simulink model "qless_forgetting_factor_16x16_nofifo"  (R2021a)
settings: Solver=FixedStepDiscrete  StartTime=0.0  StopTime=stoptime*inf  RelTol=1e-3
InitFcn:
  | qless_init_16chan_fi
undefined symbols (not defined in the file): fc, numArrayElements, physconst, srcAngles, Ts
libraries: hdlsllib x137, commfilt2 x4, commrfcorlib x3, commsync2 x3, commrflib2 x2, commrandsrc3 x2, simulink x2, phasedtxrxlib x2, commdigbbndcpm2 x1, embreciprocals x1, commdigbbndpm3 x1
(part 9 of 22)

== system qless_forgetting_factor_16x16_nofifo/MVDR_QLess_HDL/Complex Partial-Systolic Matrix Solve Using Q-less QR Decomposition with Forgetting Factor Manually Tiled n=16/Complex Partial-Systolic Q-less QR with Forgetting Factor/Complex Partial-Systolic Q-less QR with Forgetting Factor Manually tiled/Complex Partial-Systolic Q-less QR Decomposition with Forgetting Factor Section Constant pivot3/Complex Partial-Systolic Q-less QR Row Rotations/ValidIn to Ready Logic1 ==
  readyIn : Inport
  validIn : Inport  Port=2
  AND : Logic  IconShape=distinctive  AllPortsSameDT=off  OutDataTypeStr=boolean
  NOT : Logic  Operator=NOT  IconShape=distinctive  AllPortsSameDT=off  OutDataTypeStr=boolean
  readyOut : Outport  VectorParamsAs1DForOutWhenUnconnected=off
  wires:
  validIn/1 -> NOT/1
  readyIn/1 -> AND/1
  AND/1 -> readyOut/1
  NOT/1 -> AND/2

== system qless_forgetting_factor_16x16_nofifo/MVDR_QLess_HDL/Complex Partial-Systolic Matrix Solve Using Q-less QR Decomposition with Forgetting Factor Manually Tiled n=16/Complex Partial-Systolic Q-less QR with Forgetting Factor/Complex Partial-Systolic Q-less QR with Forgetting Factor Manually tiled/Complex Partial-Systolic Q-less QR Decomposition with Forgetting Factor Section Constant pivot4/Complex Partial-Systolic Q-less QR Row Rotations/Complex Partial-Systolic Q-less QR CORDIC Row Rotation ==
  x : Inport
  y : Inport  Port=2
  validIn : Inport  Port=3
  restart : Inport  Port=4
  CORDIC QR Kernel : MATLAB Function  TreatAsAtomicUnit=on
  Delay{1..3,6} (4 alike) : Delay  DelayLength=1
  State Control : StateControl  StateControl=Synchronous
  Unit Delay Enabled Synchronous1 : hdlsllib/Discrete/Unit Delay Enabled Synchronous  InitialCondition=0.0  SampleTime=-1
      settings: SourceProductBaseCode=SL
  Unit Delay Enabled Synchronous4 : hdlsllib/Discrete/Unit Delay Enabled Synchronous  InitialCondition=0.0  SampleTime=-1
      settings: SourceProductBaseCode=SL
  xOut : Outport  VectorParamsAs1DForOutWhenUnconnected=off
  yOut : Outport  Port=2  VectorParamsAs1DForOutWhenUnconnected=off
  validOut : Outport  Port=3  VectorParamsAs1DForOutWhenUnconnected=off
  ready : Outport  Port=4  VectorParamsAs1DForOutWhenUnconnected=off
  wires:
  Delay3/1 -> validOut/1
  Unit Delay Enabled Synchronous1/1 -> yOut/1
  CORDIC QR Kernel/1(xOut) -> Unit Delay Enabled Synchronous4/1
  y/1 -> Delay2/1
  x/1 -> Delay1/1
  CORDIC QR Kernel/2(yOut) -> Unit Delay Enabled Synchronous1/1
  validIn/1 -> Delay6/1
  Unit Delay Enabled Synchronous4/1 -> xOut/1
  restart/1 -> CORDIC QR Kernel/4(restart)
  CORDIC QR Kernel/3(validOut) -> Delay3/1, Unit Delay Enabled Synchronous4/2, Unit Delay Enabled Synchronous1/2
  CORDIC QR Kernel/4(ready) -> ready/1
  Delay1/1 -> CORDIC QR Kernel/1(xIn)
  Delay2/1 -> CORDIC QR Kernel/2(yIn)
  Delay6/1 -> CORDIC QR Kernel/3(validIn)

== system qless_forgetting_factor_16x16_nofifo/MVDR_QLess_HDL/Complex Partial-Systolic Matrix Solve Using Q-less QR Decomposition with Forgetting Factor Manually Tiled n=16/Complex Partial-Systolic Q-less QR with Forgetting Factor/Complex Partial-Systolic Q-less QR with Forgetting Factor Manually tiled/Complex Partial-Systolic Q-less QR Decomposition with Forgetting Factor Section Constant pivot4/Complex Partial-Systolic Q-less QR Row Rotations/Inverse CORDIC Gain1 ==
  u : Inport
  MATLAB Function : MATLAB Function  TreatAsAtomicUnit=on
  y : Outport  VectorParamsAs1DForOutWhenUnconnected=off
  wires:
  MATLAB Function/1(y) -> y/1
  u/1 -> MATLAB Function/1(u)

== system qless_forgetting_factor_16x16_nofifo/MVDR_QLess_HDL/Complex Partial-Systolic Matrix Solve Using Q-less QR Decomposition with Forgetting Factor Manually Tiled n=16/Complex Partial-Systolic Q-less QR with Forgetting Factor/Complex Partial-Systolic Q-less QR with Forgetting Factor Manually tiled/Complex Partial-Systolic Q-less QR Decomposition with Forgetting Factor Section Constant pivot4/Complex Partial-Systolic Q-less QR Row Rotations/Inverse CORDIC Gain4 ==
  u : Inport
  MATLAB Function : MATLAB Function  TreatAsAtomicUnit=on
  y : Outport  VectorParamsAs1DForOutWhenUnconnected=off
  wires:
  MATLAB Function/1(y) -> y/1
  u/1 -> MATLAB Function/1(u)

== system qless_forgetting_factor_16x16_nofifo/MVDR_QLess_HDL/Complex Partial-Systolic Matrix Solve Using Q-less QR Decomposition with Forgetting Factor Manually Tiled n=16/Complex Partial-Systolic Q-less QR with Forgetting Factor/Complex Partial-Systolic Q-less QR with Forgetting Factor Manually tiled/Complex Partial-Systolic Q-less QR Decomposition with Forgetting Factor Section Constant pivot4/Complex Partial-Systolic Q-less QR Row Rotations/Q-less QR Rotate First Element To Real1 ==
  x : Inport
  validIn : Inport  Port=2
  restart : Inport  Port=3
  Complex to Real-Imag : ComplexToRealImag
  Delay15 : Delay  DelayLength=1
  Delay9 : Delay  DelayLength=1
  Q-less QR Real Row Rotations : Subsystem  mask(QR Real Row Rotations){n=n, pivot=pivot}
      mask prompts: n "fixed:emblib:ColumnsInA"
      mask help: fixed:emblib:RowRotationsFullDescription
      mask DialogControl n Prompt: Number of columns in matrix A
  Real-Imag to Complex : RealImagToComplex
  State Control : StateControl  StateControl=Synchronous
  Unit Delay Enabled Synchronous1 : hdlsllib/Discrete/Unit Delay Enabled Synchronous  InitialCondition=0.0  SampleTime=-1
      settings: SourceProductBaseCode=SL
  Unit Delay Enabled Synchronous3 : hdlsllib/Discrete/Unit Delay Enabled Synchronous  InitialCondition=0.0  SampleTime=-1
      settings: SourceProductBaseCode=SL
  ValidIn to Ready Logic : Subsystem
  ValidIn to Ready Logic1 : Subsystem
  xOut : Outport  VectorParamsAs1DForOutWhenUnconnected=off
  validOut : Outport  Port=2  VectorParamsAs1DForOutWhenUnconnected=off
  ready : Outport  Port=3  VectorParamsAs1DForOutWhenUnconnected=off
  wires:
  Q-less QR Real Row Rotations/2(yOut) -> Real-Imag to Complex/2
  Q-less QR Real Row Rotations/1(xOut) -> Real-Imag to Complex/1
  Complex to Real-Imag/2 -> Q-less QR Real Row Rotations/2(y)
  Complex to Real-Imag/1 -> Q-less QR Real Row Rotations/1(x)
  restart/1 -> Q-less QR Real Row Rotations/4(restart)
  ValidIn to Ready Logic1/1(readyOut) -> ready/1
  ValidIn to Ready Logic/1(readyOut) -> ValidIn to Ready Logic1/1(readyIn)
  Q-less QR Real Row Rotations/4(ready) -> ValidIn to Ready Logic/1(readyIn)
  Q-less QR Real Row Rotations/3(validOut) -> Delay15/1, Unit Delay Enabled Synchronous3/2
  Delay9/1 -> ValidIn to Ready Logic/2(validIn), Q-less QR Real Row Rotations/3(validIn)
  x/1 -> Unit Delay Enabled Synchronous1/1
  validIn/1 -> ValidIn to Ready Logic1/2(validIn), Delay9/1, Unit Delay Enabled Synchronous1/2
  Delay15/1 -> validOut/1
  Unit Delay Enabled Synchronous1/1 -> Complex to Real-Imag/1
  Real-Imag to Complex/1 -> Unit Delay Enabled Synchronous3/1
  Unit Delay Enabled Synchronous3/1 -> xOut/1

== system qless_forgetting_factor_16x16_nofifo/MVDR_QLess_HDL/Complex Partial-Systolic Matrix Solve Using Q-less QR Decomposition with Forgetting Factor Manually Tiled n=16/Complex Partial-Systolic Q-less QR with Forgetting Factor/Complex Partial-Systolic Q-less QR with Forgetting Factor Manually tiled/Complex Partial-Systolic Q-less QR Decomposition with Forgetting Factor Section Constant pivot4/Complex Partial-Systolic Q-less QR Row Rotations/Set Element To Zero1 ==
  u : Inport
  Set Element To Zero : MATLAB Function  TreatAsAtomicUnit=on
  y : Outport  VectorParamsAs1DForOutWhenUnconnected=off
  wires:
  Set Element To Zero/1(y) -> y/1
  u/1 -> Set Element To Zero/1(u)

== system qless_forgetting_factor_16x16_nofifo/MVDR_QLess_HDL/Complex Partial-Systolic Matrix Solve Using Q-less QR Decomposition with Forgetting Factor Manually Tiled n=16/Complex Partial-Systolic Q-less QR with Forgetting Factor/Complex Partial-Systolic Q-less QR with Forgetting Factor Manually tiled/Complex Partial-Systolic Q-less QR Decomposition with Forgetting Factor Section Constant pivot4/Complex Partial-Systolic Q-less QR Row Rotations/ValidIn to Ready Logic ==
  readyIn : Inport
  validIn : Inport  Port=2
  AND : Logic  IconShape=distinctive  AllPortsSameDT=off  OutDataTypeStr=boolean
  NOT : Logic  Operator=NOT  IconShape=distinctive  AllPortsSameDT=off  OutDataTypeStr=boolean
  readyOut : Outport  VectorParamsAs1DForOutWhenUnconnected=off
  wires:
  validIn/1 -> NOT/1
  readyIn/1 -> AND/1
  AND/1 -> readyOut/1
  NOT/1 -> AND/2

== system qless_forgetting_factor_16x16_nofifo/MVDR_QLess_HDL/Complex Partial-Systolic Matrix Solve Using Q-less QR Decomposition with Forgetting Factor Manually Tiled n=16/Complex Partial-Systolic Q-less QR with Forgetting Factor/Complex Partial-Systolic Q-less QR with Forgetting Factor Manually tiled/Complex Partial-Systolic Q-less QR Decomposition with Forgetting Factor Section Constant pivot4/Complex Partial-Systolic Q-less QR Row Rotations/ValidIn to Ready Logic1 ==
  readyIn : Inport
  validIn : Inport  Port=2
  AND : Logic  IconShape=distinctive  AllPortsSameDT=off  OutDataTypeStr=boolean
  NOT : Logic  Operator=NOT  IconShape=distinctive  AllPortsSameDT=off  OutDataTypeStr=boolean
  readyOut : Outport  VectorParamsAs1DForOutWhenUnconnected=off
  wires:
  validIn/1 -> NOT/1
  readyIn/1 -> AND/1
  AND/1 -> readyOut/1
  NOT/1 -> AND/2

== system qless_forgetting_factor_16x16_nofifo/MVDR_QLess_HDL/Complex Partial-Systolic Matrix Solve Using Q-less QR Decomposition with Forgetting Factor Manually Tiled n=16/Complex Partial-Systolic Q-less QR with Forgetting Factor/Complex Partial-Systolic Q-less QR with Forgetting Factor Manually tiled/Complex Partial-Systolic Q-less QR Decomposition with Forgetting Factor Section Constant pivot5/Complex Partial-Systolic Q-less QR Row Rotations/Complex Partial-Systolic Q-less QR CORDIC Row Rotation ==
  x : Inport
  y : Inport  Port=2
  validIn : Inport  Port=3
  restart : Inport  Port=4
  CORDIC QR Kernel : MATLAB Function  TreatAsAtomicUnit=on
  Delay{1..3,6} (4 alike) : Delay  DelayLength=1
  State Control : StateControl  StateControl=Synchronous
  Unit Delay Enabled Synchronous1 : hdlsllib/Discrete/Unit Delay Enabled Synchronous  InitialCondition=0.0  SampleTime=-1
      settings: SourceProductBaseCode=SL
  Unit Delay Enabled Synchronous4 : hdlsllib/Discrete/Unit Delay Enabled Synchronous  InitialCondition=0.0  SampleTime=-1
      settings: SourceProductBaseCode=SL
  xOut : Outport  VectorParamsAs1DForOutWhenUnconnected=off
  yOut : Outport  Port=2  VectorParamsAs1DForOutWhenUnconnected=off
  validOut : Outport  Port=3  VectorParamsAs1DForOutWhenUnconnected=off
  ready : Outport  Port=4  VectorParamsAs1DForOutWhenUnconnected=off
  wires:
  Delay3/1 -> validOut/1
  Unit Delay Enabled Synchronous1/1 -> yOut/1
  CORDIC QR Kernel/1(xOut) -> Unit Delay Enabled Synchronous4/1
  y/1 -> Delay2/1
  x/1 -> Delay1/1
  CORDIC QR Kernel/2(yOut) -> Unit Delay Enabled Synchronous1/1
  validIn/1 -> Delay6/1
  Unit Delay Enabled Synchronous4/1 -> xOut/1
  restart/1 -> CORDIC QR Kernel/4(restart)
  CORDIC QR Kernel/3(validOut) -> Delay3/1, Unit Delay Enabled Synchronous4/2, Unit Delay Enabled Synchronous1/2
  CORDIC QR Kernel/4(ready) -> ready/1
  Delay1/1 -> CORDIC QR Kernel/1(xIn)
  Delay2/1 -> CORDIC QR Kernel/2(yIn)
  Delay6/1 -> CORDIC QR Kernel/3(validIn)

== system qless_forgetting_factor_16x16_nofifo/MVDR_QLess_HDL/Complex Partial-Systolic Matrix Solve Using Q-less QR Decomposition with Forgetting Factor Manually Tiled n=16/Complex Partial-Systolic Q-less QR with Forgetting Factor/Complex Partial-Systolic Q-less QR with Forgetting Factor Manually tiled/Complex Partial-Systolic Q-less QR Decomposition with Forgetting Factor Section Constant pivot5/Complex Partial-Systolic Q-less QR Row Rotations/Inverse CORDIC Gain1 ==
  u : Inport
  MATLAB Function : MATLAB Function  TreatAsAtomicUnit=on
  y : Outport  VectorParamsAs1DForOutWhenUnconnected=off
  wires:
  MATLAB Function/1(y) -> y/1
  u/1 -> MATLAB Function/1(u)

== system qless_forgetting_factor_16x16_nofifo/MVDR_QLess_HDL/Complex Partial-Systolic Matrix Solve Using Q-less QR Decomposition with Forgetting Factor Manually Tiled n=16/Complex Partial-Systolic Q-less QR with Forgetting Factor/Complex Partial-Systolic Q-less QR with Forgetting Factor Manually tiled/Complex Partial-Systolic Q-less QR Decomposition with Forgetting Factor Section Constant pivot5/Complex Partial-Systolic Q-less QR Row Rotations/Inverse CORDIC Gain4 ==
  u : Inport
  MATLAB Function : MATLAB Function  TreatAsAtomicUnit=on
  y : Outport  VectorParamsAs1DForOutWhenUnconnected=off
  wires:
  MATLAB Function/1(y) -> y/1
  u/1 -> MATLAB Function/1(u)

== system qless_forgetting_factor_16x16_nofifo/MVDR_QLess_HDL/Complex Partial-Systolic Matrix Solve Using Q-less QR Decomposition with Forgetting Factor Manually Tiled n=16/Complex Partial-Systolic Q-less QR with Forgetting Factor/Complex Partial-Systolic Q-less QR with Forgetting Factor Manually tiled/Complex Partial-Systolic Q-less QR Decomposition with Forgetting Factor Section Constant pivot5/Complex Partial-Systolic Q-less QR Row Rotations/Q-less QR Rotate First Element To Real1 ==
  x : Inport
  validIn : Inport  Port=2
  restart : Inport  Port=3
  Complex to Real-Imag : ComplexToRealImag
  Delay15 : Delay  DelayLength=1
  Delay9 : Delay  DelayLength=1
  Q-less QR Real Row Rotations : Subsystem  mask(QR Real Row Rotations){n=n, pivot=pivot}
      mask prompts: n "fixed:emblib:ColumnsInA"
      mask help: fixed:emblib:RowRotationsFullDescription
      mask DialogControl n Prompt: Number of columns in matrix A
  Real-Imag to Complex : RealImagToComplex
  State Control : StateControl  StateControl=Synchronous
  Unit Delay Enabled Synchronous1 : hdlsllib/Discrete/Unit Delay Enabled Synchronous  InitialCondition=0.0  SampleTime=-1
      settings: SourceProductBaseCode=SL
  Unit Delay Enabled Synchronous3 : hdlsllib/Discrete/Unit Delay Enabled Synchronous  InitialCondition=0.0  SampleTime=-1
      settings: SourceProductBaseCode=SL
  ValidIn to Ready Logic : Subsystem
  ValidIn to Ready Logic1 : Subsystem
  xOut : Outport  VectorParamsAs1DForOutWhenUnconnected=off
  validOut : Outport  Port=2  VectorParamsAs1DForOutWhenUnconnected=off
  ready : Outport  Port=3  VectorParamsAs1DForOutWhenUnconnected=off
  wires:
  Q-less QR Real Row Rotations/2(yOut) -> Real-Imag to Complex/2
  Q-less QR Real Row Rotations/1(xOut) -> Real-Imag to Complex/1
  Complex to Real-Imag/2 -> Q-less QR Real Row Rotations/2(y)
  Complex to Real-Imag/1 -> Q-less QR Real Row Rotations/1(x)
  restart/1 -> Q-less QR Real Row Rotations/4(restart)
  ValidIn to Ready Logic1/1(readyOut) -> ready/1
  ValidIn to Ready Logic/1(readyOut) -> ValidIn to Ready Logic1/1(readyIn)
  Q-less QR Real Row Rotations/4(ready) -> ValidIn to Ready Logic/1(readyIn)
  Q-less QR Real Row Rotations/3(validOut) -> Delay15/1, Unit Delay Enabled Synchronous3/2
  Delay9/1 -> ValidIn to Ready Logic/2(validIn), Q-less QR Real Row Rotations/3(validIn)
  x/1 -> Unit Delay Enabled Synchronous1/1
  validIn/1 -> ValidIn to Ready Logic1/2(validIn), Delay9/1, Unit Delay Enabled Synchronous1/2
  Delay15/1 -> validOut/1
  Unit Delay Enabled Synchronous1/1 -> Complex to Real-Imag/1
  Real-Imag to Complex/1 -> Unit Delay Enabled Synchronous3/1
  Unit Delay Enabled Synchronous3/1 -> xOut/1

== system qless_forgetting_factor_16x16_nofifo/MVDR_QLess_HDL/Complex Partial-Systolic Matrix Solve Using Q-less QR Decomposition with Forgetting Factor Manually Tiled n=16/Complex Partial-Systolic Q-less QR with Forgetting Factor/Complex Partial-Systolic Q-less QR with Forgetting Factor Manually tiled/Complex Partial-Systolic Q-less QR Decomposition with Forgetting Factor Section Constant pivot5/Complex Partial-Systolic Q-less QR Row Rotations/Set Element To Zero1 ==
  u : Inport
  Set Element To Zero : MATLAB Function  TreatAsAtomicUnit=on
  y : Outport  VectorParamsAs1DForOutWhenUnconnected=off
  wires:
  Set Element To Zero/1(y) -> y/1
  u/1 -> Set Element To Zero/1(u)

== system qless_forgetting_factor_16x16_nofifo/MVDR_QLess_HDL/Complex Partial-Systolic Matrix Solve Using Q-less QR Decomposition with Forgetting Factor Manually Tiled n=16/Complex Partial-Systolic Q-less QR with Forgetting Factor/Complex Partial-Systolic Q-less QR with Forgetting Factor Manually tiled/Complex Partial-Systolic Q-less QR Decomposition with Forgetting Factor Section Constant pivot5/Complex Partial-Systolic Q-less QR Row Rotations/ValidIn to Ready Logic ==
  readyIn : Inport
  validIn : Inport  Port=2
  AND : Logic  IconShape=distinctive  AllPortsSameDT=off  OutDataTypeStr=boolean
  NOT : Logic  Operator=NOT  IconShape=distinctive  AllPortsSameDT=off  OutDataTypeStr=boolean
  readyOut : Outport  VectorParamsAs1DForOutWhenUnconnected=off
  wires:
  validIn/1 -> NOT/1
  readyIn/1 -> AND/1
  AND/1 -> readyOut/1
  NOT/1 -> AND/2

== system qless_forgetting_factor_16x16_nofifo/MVDR_QLess_HDL/Complex Partial-Systolic Matrix Solve Using Q-less QR Decomposition with Forgetting Factor Manually Tiled n=16/Complex Partial-Systolic Q-less QR with Forgetting Factor/Complex Partial-Systolic Q-less QR with Forgetting Factor Manually tiled/Complex Partial-Systolic Q-less QR Decomposition with Forgetting Factor Section Constant pivot5/Complex Partial-Systolic Q-less QR Row Rotations/ValidIn to Ready Logic1 ==
  readyIn : Inport
  validIn : Inport  Port=2
  AND : Logic  IconShape=distinctive  AllPortsSameDT=off  OutDataTypeStr=boolean
  NOT : Logic  Operator=NOT  IconShape=distinctive  AllPortsSameDT=off  OutDataTypeStr=boolean
  readyOut : Outport  VectorParamsAs1DForOutWhenUnconnected=off
  wires:
  validIn/1 -> NOT/1
  readyIn/1 -> AND/1
  AND/1 -> readyOut/1
  NOT/1 -> AND/2

== system qless_forgetting_factor_16x16_nofifo/MVDR_QLess_HDL/Complex Partial-Systolic Matrix Solve Using Q-less QR Decomposition with Forgetting Factor Manually Tiled n=16/Complex Partial-Systolic Q-less QR with Forgetting Factor/Complex Partial-Systolic Q-less QR with Forgetting Factor Manually tiled/Complex Partial-Systolic Q-less QR Decomposition with Forgetting Factor Section Constant pivot6/Complex Partial-Systolic Q-less QR Row Rotations/Complex Partial-Systolic Q-less QR CORDIC Row Rotation ==
  x : Inport
  y : Inport  Port=2
  validIn : Inport  Port=3
  restart : Inport  Port=4
  CORDIC QR Kernel : MATLAB Function  TreatAsAtomicUnit=on
  Delay{1..3,6} (4 alike) : Delay  DelayLength=1
  State Control : StateControl  StateControl=Synchronous
  Unit Delay Enabled Synchronous1 : hdlsllib/Discrete/Unit Delay Enabled Synchronous  InitialCondition=0.0  SampleTime=-1
      settings: SourceProductBaseCode=SL
  Unit Delay Enabled Synchronous4 : hdlsllib/Discrete/Unit Delay Enabled Synchronous  InitialCondition=0.0  SampleTime=-1
      settings: SourceProductBaseCode=SL
  xOut : Outport  VectorParamsAs1DForOutWhenUnconnected=off
  yOut : Outport  Port=2  VectorParamsAs1DForOutWhenUnconnected=off
  validOut : Outport  Port=3  VectorParamsAs1DForOutWhenUnconnected=off
  ready : Outport  Port=4  VectorParamsAs1DForOutWhenUnconnected=off
  wires:
  Delay3/1 -> validOut/1
  Unit Delay Enabled Synchronous1/1 -> yOut/1
  CORDIC QR Kernel/1(xOut) -> Unit Delay Enabled Synchronous4/1
  y/1 -> Delay2/1
  x/1 -> Delay1/1
  CORDIC QR Kernel/2(yOut) -> Unit Delay Enabled Synchronous1/1
  validIn/1 -> Delay6/1
  Unit Delay Enabled Synchronous4/1 -> xOut/1
  restart/1 -> CORDIC QR Kernel/4(restart)
  CORDIC QR Kernel/3(validOut) -> Delay3/1, Unit Delay Enabled Synchronous4/2, Unit Delay Enabled Synchronous1/2
  CORDIC QR Kernel/4(ready) -> ready/1
  Delay1/1 -> CORDIC QR Kernel/1(xIn)
  Delay2/1 -> CORDIC QR Kernel/2(yIn)
  Delay6/1 -> CORDIC QR Kernel/3(validIn)

== system qless_forgetting_factor_16x16_nofifo/MVDR_QLess_HDL/Complex Partial-Systolic Matrix Solve Using Q-less QR Decomposition with Forgetting Factor Manually Tiled n=16/Complex Partial-Systolic Q-less QR with Forgetting Factor/Complex Partial-Systolic Q-less QR with Forgetting Factor Manually tiled/Complex Partial-Systolic Q-less QR Decomposition with Forgetting Factor Section Constant pivot6/Complex Partial-Systolic Q-less QR Row Rotations/Inverse CORDIC Gain1 ==
  u : Inport
  MATLAB Function : MATLAB Function  TreatAsAtomicUnit=on
  y : Outport  VectorParamsAs1DForOutWhenUnconnected=off
  wires:
  MATLAB Function/1(y) -> y/1
  u/1 -> MATLAB Function/1(u)

== system qless_forgetting_factor_16x16_nofifo/MVDR_QLess_HDL/Complex Partial-Systolic Matrix Solve Using Q-less QR Decomposition with Forgetting Factor Manually Tiled n=16/Complex Partial-Systolic Q-less QR with Forgetting Factor/Complex Partial-Systolic Q-less QR with Forgetting Factor Manually tiled/Complex Partial-Systolic Q-less QR Decomposition with Forgetting Factor Section Constant pivot6/Complex Partial-Systolic Q-less QR Row Rotations/Inverse CORDIC Gain4 ==
  u : Inport
  MATLAB Function : MATLAB Function  TreatAsAtomicUnit=on
  y : Outport  VectorParamsAs1DForOutWhenUnconnected=off
  wires:
  MATLAB Function/1(y) -> y/1
  u/1 -> MATLAB Function/1(u)

== system qless_forgetting_factor_16x16_nofifo/MVDR_QLess_HDL/Complex Partial-Systolic Matrix Solve Using Q-less QR Decomposition with Forgetting Factor Manually Tiled n=16/Complex Partial-Systolic Q-less QR with Forgetting Factor/Complex Partial-Systolic Q-less QR with Forgetting Factor Manually tiled/Complex Partial-Systolic Q-less QR Decomposition with Forgetting Factor Section Constant pivot6/Complex Partial-Systolic Q-less QR Row Rotations/Q-less QR Rotate First Element To Real1 ==
  x : Inport
  validIn : Inport  Port=2
  restart : Inport  Port=3
  Complex to Real-Imag : ComplexToRealImag
  Delay15 : Delay  DelayLength=1
  Delay9 : Delay  DelayLength=1
  Q-less QR Real Row Rotations : Subsystem  mask(QR Real Row Rotations){n=n, pivot=pivot}
      mask prompts: n "fixed:emblib:ColumnsInA"
      mask help: fixed:emblib:RowRotationsFullDescription
      mask DialogControl n Prompt: Number of columns in matrix A
  Real-Imag to Complex : RealImagToComplex
  State Control : StateControl  StateControl=Synchronous
  Unit Delay Enabled Synchronous1 : hdlsllib/Discrete/Unit Delay Enabled Synchronous  InitialCondition=0.0  SampleTime=-1
      settings: SourceProductBaseCode=SL
  Unit Delay Enabled Synchronous3 : hdlsllib/Discrete/Unit Delay Enabled Synchronous  InitialCondition=0.0  SampleTime=-1
      settings: SourceProductBaseCode=SL
  ValidIn to Ready Logic : Subsystem
  ValidIn to Ready Logic1 : Subsystem
  xOut : Outport  VectorParamsAs1DForOutWhenUnconnected=off
  validOut : Outport  Port=2  VectorParamsAs1DForOutWhenUnconnected=off
  ready : Outport  Port=3  VectorParamsAs1DForOutWhenUnconnected=off
  wires:
  Q-less QR Real Row Rotations/2(yOut) -> Real-Imag to Complex/2
  Q-less QR Real Row Rotations/1(xOut) -> Real-Imag to Complex/1
  Complex to Real-Imag/2 -> Q-less QR Real Row Rotations/2(y)
  Complex to Real-Imag/1 -> Q-less QR Real Row Rotations/1(x)
  restart/1 -> Q-less QR Real Row Rotations/4(restart)
  ValidIn to Ready Logic1/1(readyOut) -> ready/1
  ValidIn to Ready Logic/1(readyOut) -> ValidIn to Ready Logic1/1(readyIn)
  Q-less QR Real Row Rotations/4(ready) -> ValidIn to Ready Logic/1(readyIn)
  Q-less QR Real Row Rotations/3(validOut) -> Delay15/1, Unit Delay Enabled Synchronous3/2
  Delay9/1 -> ValidIn to Ready Logic/2(validIn), Q-less QR Real Row Rotations/3(validIn)
  x/1 -> Unit Delay Enabled Synchronous1/1
  validIn/1 -> ValidIn to Ready Logic1/2(validIn), Delay9/1, Unit Delay Enabled Synchronous1/2
  Delay15/1 -> validOut/1
  Unit Delay Enabled Synchronous1/1 -> Complex to Real-Imag/1
  Real-Imag to Complex/1 -> Unit Delay Enabled Synchronous3/1
  Unit Delay Enabled Synchronous3/1 -> xOut/1

== system qless_forgetting_factor_16x16_nofifo/MVDR_QLess_HDL/Complex Partial-Systolic Matrix Solve Using Q-less QR Decomposition with Forgetting Factor Manually Tiled n=16/Complex Partial-Systolic Q-less QR with Forgetting Factor/Complex Partial-Systolic Q-less QR with Forgetting Factor Manually tiled/Complex Partial-Systolic Q-less QR Decomposition with Forgetting Factor Section Constant pivot6/Complex Partial-Systolic Q-less QR Row Rotations/Set Element To Zero1 ==
  u : Inport
  Set Element To Zero : MATLAB Function  TreatAsAtomicUnit=on
  y : Outport  VectorParamsAs1DForOutWhenUnconnected=off
  wires:
  Set Element To Zero/1(y) -> y/1
  u/1 -> Set Element To Zero/1(u)

== system qless_forgetting_factor_16x16_nofifo/MVDR_QLess_HDL/Complex Partial-Systolic Matrix Solve Using Q-less QR Decomposition with Forgetting Factor Manually Tiled n=16/Complex Partial-Systolic Q-less QR with Forgetting Factor/Complex Partial-Systolic Q-less QR with Forgetting Factor Manually tiled/Complex Partial-Systolic Q-less QR Decomposition with Forgetting Factor Section Constant pivot6/Complex Partial-Systolic Q-less QR Row Rotations/ValidIn to Ready Logic ==
  readyIn : Inport
  validIn : Inport  Port=2
  AND : Logic  IconShape=distinctive  AllPortsSameDT=off  OutDataTypeStr=boolean
  NOT : Logic  Operator=NOT  IconShape=distinctive  AllPortsSameDT=off  OutDataTypeStr=boolean
  readyOut : Outport  VectorParamsAs1DForOutWhenUnconnected=off
  wires:
  validIn/1 -> NOT/1
  readyIn/1 -> AND/1
  AND/1 -> readyOut/1
  NOT/1 -> AND/2

== system qless_forgetting_factor_16x16_nofifo/MVDR_QLess_HDL/Complex Partial-Systolic Matrix Solve Using Q-less QR Decomposition with Forgetting Factor Manually Tiled n=16/Complex Partial-Systolic Q-less QR with Forgetting Factor/Complex Partial-Systolic Q-less QR with Forgetting Factor Manually tiled/Complex Partial-Systolic Q-less QR Decomposition with Forgetting Factor Section Constant pivot6/Complex Partial-Systolic Q-less QR Row Rotations/ValidIn to Ready Logic1 ==
  readyIn : Inport
  validIn : Inport  Port=2
  AND : Logic  IconShape=distinctive  AllPortsSameDT=off  OutDataTypeStr=boolean
  NOT : Logic  Operator=NOT  IconShape=distinctive  AllPortsSameDT=off  OutDataTypeStr=boolean
  readyOut : Outport  VectorParamsAs1DForOutWhenUnconnected=off
  wires:
  validIn/1 -> NOT/1
  readyIn/1 -> AND/1
  AND/1 -> readyOut/1
  NOT/1 -> AND/2

== system qless_forgetting_factor_16x16_nofifo/MVDR_QLess_HDL/Complex Partial-Systolic Matrix Solve Using Q-less QR Decomposition with Forgetting Factor Manually Tiled n=16/Complex Partial-Systolic Q-less QR with Forgetting Factor/Complex Partial-Systolic Q-less QR with Forgetting Factor Manually tiled/Complex Partial-Systolic Q-less QR Decomposition with Forgetting Factor Section Constant pivot7/Complex Partial-Systolic Q-less QR Row Rotations/Complex Partial-Systolic Q-less QR CORDIC Row Rotation ==
  x : Inport
  y : Inport  Port=2
  validIn : Inport  Port=3
  restart : Inport  Port=4
  CORDIC QR Kernel : MATLAB Function  TreatAsAtomicUnit=on
  Delay{1..3,6} (4 alike) : Delay  DelayLength=1
  State Control : StateControl  StateControl=Synchronous
  Unit Delay Enabled Synchronous1 : hdlsllib/Discrete/Unit Delay Enabled Synchronous  InitialCondition=0.0  SampleTime=-1
      settings: SourceProductBaseCode=SL
  Unit Delay Enabled Synchronous4 : hdlsllib/Discrete/Unit Delay Enabled Synchronous  InitialCondition=0.0  SampleTime=-1
      settings: SourceProductBaseCode=SL
  xOut : Outport  VectorParamsAs1DForOutWhenUnconnected=off
  yOut : Outport  Port=2  VectorParamsAs1DForOutWhenUnconnected=off
  validOut : Outport  Port=3  VectorParamsAs1DForOutWhenUnconnected=off
  ready : Outport  Port=4  VectorParamsAs1DForOutWhenUnconnected=off
  wires:
  Delay3/1 -> validOut/1
  Unit Delay Enabled Synchronous1/1 -> yOut/1
  CORDIC QR Kernel/1(xOut) -> Unit Delay Enabled Synchronous4/1
  y/1 -> Delay2/1
  x/1 -> Delay1/1
  CORDIC QR Kernel/2(yOut) -> Unit Delay Enabled Synchronous1/1
  validIn/1 -> Delay6/1
  Unit Delay Enabled Synchronous4/1 -> xOut/1
  restart/1 -> CORDIC QR Kernel/4(restart)
  CORDIC QR Kernel/3(validOut) -> Delay3/1, Unit Delay Enabled Synchronous4/2, Unit Delay Enabled Synchronous1/2
  CORDIC QR Kernel/4(ready) -> ready/1
  Delay1/1 -> CORDIC QR Kernel/1(xIn)
  Delay2/1 -> CORDIC QR Kernel/2(yIn)
  Delay6/1 -> CORDIC QR Kernel/3(validIn)

== system qless_forgetting_factor_16x16_nofifo/MVDR_QLess_HDL/Complex Partial-Systolic Matrix Solve Using Q-less QR Decomposition with Forgetting Factor Manually Tiled n=16/Complex Partial-Systolic Q-less QR with Forgetting Factor/Complex Partial-Systolic Q-less QR with Forgetting Factor Manually tiled/Complex Partial-Systolic Q-less QR Decomposition with Forgetting Factor Section Constant pivot7/Complex Partial-Systolic Q-less QR Row Rotations/Inverse CORDIC Gain1 ==
  u : Inport
  MATLAB Function : MATLAB Function  TreatAsAtomicUnit=on
  y : Outport  VectorParamsAs1DForOutWhenUnconnected=off
  wires:
  MATLAB Function/1(y) -> y/1
  u/1 -> MATLAB Function/1(u)

== system qless_forgetting_factor_16x16_nofifo/MVDR_QLess_HDL/Complex Partial-Systolic Matrix Solve Using Q-less QR Decomposition with Forgetting Factor Manually Tiled n=16/Complex Partial-Systolic Q-less QR with Forgetting Factor/Complex Partial-Systolic Q-less QR with Forgetting Factor Manually tiled/Complex Partial-Systolic Q-less QR Decomposition with Forgetting Factor Section Constant pivot7/Complex Partial-Systolic Q-less QR Row Rotations/Inverse CORDIC Gain4 ==
  u : Inport
  MATLAB Function : MATLAB Function  TreatAsAtomicUnit=on
  y : Outport  VectorParamsAs1DForOutWhenUnconnected=off
  wires:
  MATLAB Function/1(y) -> y/1
  u/1 -> MATLAB Function/1(u)

== system qless_forgetting_factor_16x16_nofifo/MVDR_QLess_HDL/Complex Partial-Systolic Matrix Solve Using Q-less QR Decomposition with Forgetting Factor Manually Tiled n=16/Complex Partial-Systolic Q-less QR with Forgetting Factor/Complex Partial-Systolic Q-less QR with Forgetting Factor Manually tiled/Complex Partial-Systolic Q-less QR Decomposition with Forgetting Factor Section Constant pivot7/Complex Partial-Systolic Q-less QR Row Rotations/Q-less QR Rotate First Element To Real1 ==
  x : Inport
  validIn : Inport  Port=2
  restart : Inport  Port=3
  Complex to Real-Imag : ComplexToRealImag
  Delay15 : Delay  DelayLength=1
  Delay9 : Delay  DelayLength=1
  Q-less QR Real Row Rotations : Subsystem  mask(QR Real Row Rotations){n=n, pivot=pivot}
      mask prompts: n "fixed:emblib:ColumnsInA"
      mask help: fixed:emblib:RowRotationsFullDescription
      mask DialogControl n Prompt: Number of columns in matrix A
  Real-Imag to Complex : RealImagToComplex
  State Control : StateControl  StateControl=Synchronous
  Unit Delay Enabled Synchronous1 : hdlsllib/Discrete/Unit Delay Enabled Synchronous  InitialCondition=0.0  SampleTime=-1
      settings: SourceProductBaseCode=SL
  Unit Delay Enabled Synchronous3 : hdlsllib/Discrete/Unit Delay Enabled Synchronous  InitialCondition=0.0  SampleTime=-1
      settings: SourceProductBaseCode=SL
  ValidIn to Ready Logic : Subsystem
  ValidIn to Ready Logic1 : Subsystem
  xOut : Outport  VectorParamsAs1DForOutWhenUnconnected=off
  validOut : Outport  Port=2  VectorParamsAs1DForOutWhenUnconnected=off
  ready : Outport  Port=3  VectorParamsAs1DForOutWhenUnconnected=off
  wires:
  Q-less QR Real Row Rotations/2(yOut) -> Real-Imag to Complex/2
  Q-less QR Real Row Rotations/1(xOut) -> Real-Imag to Complex/1
  Complex to Real-Imag/2 -> Q-less QR Real Row Rotations/2(y)
  Complex to Real-Imag/1 -> Q-less QR Real Row Rotations/1(x)
  restart/1 -> Q-less QR Real Row Rotations/4(restart)
  ValidIn to Ready Logic1/1(readyOut) -> ready/1
  ValidIn to Ready Logic/1(readyOut) -> ValidIn to Ready Logic1/1(readyIn)
  Q-less QR Real Row Rotations/4(ready) -> ValidIn to Ready Logic/1(readyIn)
  Q-less QR Real Row Rotations/3(validOut) -> Delay15/1, Unit Delay Enabled Synchronous3/2
  Delay9/1 -> ValidIn to Ready Logic/2(validIn), Q-less QR Real Row Rotations/3(validIn)
  x/1 -> Unit Delay Enabled Synchronous1/1
  validIn/1 -> ValidIn to Ready Logic1/2(validIn), Delay9/1, Unit Delay Enabled Synchronous1/2
  Delay15/1 -> validOut/1
  Unit Delay Enabled Synchronous1/1 -> Complex to Real-Imag/1
  Real-Imag to Complex/1 -> Unit Delay Enabled Synchronous3/1
  Unit Delay Enabled Synchronous3/1 -> xOut/1

== system qless_forgetting_factor_16x16_nofifo/MVDR_QLess_HDL/Complex Partial-Systolic Matrix Solve Using Q-less QR Decomposition with Forgetting Factor Manually Tiled n=16/Complex Partial-Systolic Q-less QR with Forgetting Factor/Complex Partial-Systolic Q-less QR with Forgetting Factor Manually tiled/Complex Partial-Systolic Q-less QR Decomposition with Forgetting Factor Section Constant pivot7/Complex Partial-Systolic Q-less QR Row Rotations/Set Element To Zero1 ==
  u : Inport
  Set Element To Zero : MATLAB Function  TreatAsAtomicUnit=on
  y : Outport  VectorParamsAs1DForOutWhenUnconnected=off
  wires:
  Set Element To Zero/1(y) -> y/1
  u/1 -> Set Element To Zero/1(u)

== system qless_forgetting_factor_16x16_nofifo/MVDR_QLess_HDL/Complex Partial-Systolic Matrix Solve Using Q-less QR Decomposition with Forgetting Factor Manually Tiled n=16/Complex Partial-Systolic Q-less QR with Forgetting Factor/Complex Partial-Systolic Q-less QR with Forgetting Factor Manually tiled/Complex Partial-Systolic Q-less QR Decomposition with Forgetting Factor Section Constant pivot7/Complex Partial-Systolic Q-less QR Row Rotations/ValidIn to Ready Logic ==
  readyIn : Inport
  validIn : Inport  Port=2
  AND : Logic  IconShape=distinctive  AllPortsSameDT=off  OutDataTypeStr=boolean
  NOT : Logic  Operator=NOT  IconShape=distinctive  AllPortsSameDT=off  OutDataTypeStr=boolean
  readyOut : Outport  VectorParamsAs1DForOutWhenUnconnected=off
  wires:
  validIn/1 -> NOT/1
  readyIn/1 -> AND/1
  AND/1 -> readyOut/1
  NOT/1 -> AND/2

== system qless_forgetting_factor_16x16_nofifo/MVDR_QLess_HDL/Complex Partial-Systolic Matrix Solve Using Q-less QR Decomposition with Forgetting Factor Manually Tiled n=16/Complex Partial-Systolic Q-less QR with Forgetting Factor/Complex Partial-Systolic Q-less QR with Forgetting Factor Manually tiled/Complex Partial-Systolic Q-less QR Decomposition with Forgetting Factor Section Constant pivot7/Complex Partial-Systolic Q-less QR Row Rotations/ValidIn to Ready Logic1 ==
  readyIn : Inport
  validIn : Inport  Port=2
  AND : Logic  IconShape=distinctive  AllPortsSameDT=off  OutDataTypeStr=boolean
  NOT : Logic  Operator=NOT  IconShape=distinctive  AllPortsSameDT=off  OutDataTypeStr=boolean
  readyOut : Outport  VectorParamsAs1DForOutWhenUnconnected=off
  wires:
  validIn/1 -> NOT/1
  readyIn/1 -> AND/1
  AND/1 -> readyOut/1
  NOT/1 -> AND/2

== system qless_forgetting_factor_16x16_nofifo/MVDR_QLess_HDL/Complex Partial-Systolic Matrix Solve Using Q-less QR Decomposition with Forgetting Factor Manually Tiled n=16/Complex Partial-Systolic Q-less QR with Forgetting Factor/Complex Partial-Systolic Q-less QR with Forgetting Factor Manually tiled/Complex Partial-Systolic Q-less QR Decomposition with Forgetting Factor Section Constant pivot8/Complex Partial-Systolic Q-less QR Row Rotations/Complex Partial-Systolic Q-less QR CORDIC Row Rotation ==
  x : Inport
  y : Inport  Port=2
  validIn : Inport  Port=3
  restart : Inport  Port=4
  CORDIC QR Kernel : MATLAB Function  TreatAsAtomicUnit=on
  Delay{1..3,6} (4 alike) : Delay  DelayLength=1
  State Control : StateControl  StateControl=Synchronous
  Unit Delay Enabled Synchronous1 : hdlsllib/Discrete/Unit Delay Enabled Synchronous  InitialCondition=0.0  SampleTime=-1
      settings: SourceProductBaseCode=SL
  Unit Delay Enabled Synchronous4 : hdlsllib/Discrete/Unit Delay Enabled Synchronous  InitialCondition=0.0  SampleTime=-1
      settings: SourceProductBaseCode=SL
  xOut : Outport  VectorParamsAs1DForOutWhenUnconnected=off
  yOut : Outport  Port=2  VectorParamsAs1DForOutWhenUnconnected=off
  validOut : Outport  Port=3  VectorParamsAs1DForOutWhenUnconnected=off
  ready : Outport  Port=4  VectorParamsAs1DForOutWhenUnconnected=off
  wires:
  Delay3/1 -> validOut/1
  Unit Delay Enabled Synchronous1/1 -> yOut/1
  CORDIC QR Kernel/1(xOut) -> Unit Delay Enabled Synchronous4/1
  y/1 -> Delay2/1
  x/1 -> Delay1/1
  CORDIC QR Kernel/2(yOut) -> Unit Delay Enabled Synchronous1/1
  validIn/1 -> Delay6/1
  Unit Delay Enabled Synchronous4/1 -> xOut/1
  restart/1 -> CORDIC QR Kernel/4(restart)
  CORDIC QR Kernel/3(validOut) -> Delay3/1, Unit Delay Enabled Synchronous4/2, Unit Delay Enabled Synchronous1/2
  CORDIC QR Kernel/4(ready) -> ready/1
  Delay1/1 -> CORDIC QR Kernel/1(xIn)
  Delay2/1 -> CORDIC QR Kernel/2(yIn)
  Delay6/1 -> CORDIC QR Kernel/3(validIn)

== system qless_forgetting_factor_16x16_nofifo/MVDR_QLess_HDL/Complex Partial-Systolic Matrix Solve Using Q-less QR Decomposition with Forgetting Factor Manually Tiled n=16/Complex Partial-Systolic Q-less QR with Forgetting Factor/Complex Partial-Systolic Q-less QR with Forgetting Factor Manually tiled/Complex Partial-Systolic Q-less QR Decomposition with Forgetting Factor Section Constant pivot8/Complex Partial-Systolic Q-less QR Row Rotations/Inverse CORDIC Gain1 ==
  u : Inport
  MATLAB Function : MATLAB Function  TreatAsAtomicUnit=on
  y : Outport  VectorParamsAs1DForOutWhenUnconnected=off
  wires:
  MATLAB Function/1(y) -> y/1
  u/1 -> MATLAB Function/1(u)

== system qless_forgetting_factor_16x16_nofifo/MVDR_QLess_HDL/Complex Partial-Systolic Matrix Solve Using Q-less QR Decomposition with Forgetting Factor Manually Tiled n=16/Complex Partial-Systolic Q-less QR with Forgetting Factor/Complex Partial-Systolic Q-less QR with Forgetting Factor Manually tiled/Complex Partial-Systolic Q-less QR Decomposition with Forgetting Factor Section Constant pivot8/Complex Partial-Systolic Q-less QR Row Rotations/Inverse CORDIC Gain4 ==
  u : Inport
  MATLAB Function : MATLAB Function  TreatAsAtomicUnit=on
  y : Outport  VectorParamsAs1DForOutWhenUnconnected=off
  wires:
  MATLAB Function/1(y) -> y/1
  u/1 -> MATLAB Function/1(u)

== system qless_forgetting_factor_16x16_nofifo/MVDR_QLess_HDL/Complex Partial-Systolic Matrix Solve Using Q-less QR Decomposition with Forgetting Factor Manually Tiled n=16/Complex Partial-Systolic Q-less QR with Forgetting Factor/Complex Partial-Systolic Q-less QR with Forgetting Factor Manually tiled/Complex Partial-Systolic Q-less QR Decomposition with Forgetting Factor Section Constant pivot8/Complex Partial-Systolic Q-less QR Row Rotations/Q-less QR Rotate First Element To Real1 ==
  x : Inport
  validIn : Inport  Port=2
  restart : Inport  Port=3
  Complex to Real-Imag : ComplexToRealImag
  Delay15 : Delay  DelayLength=1
  Delay9 : Delay  DelayLength=1
  Q-less QR Real Row Rotations : Subsystem  mask(QR Real Row Rotations){n=n, pivot=pivot}
      mask prompts: n "fixed:emblib:ColumnsInA"
      mask help: fixed:emblib:RowRotationsFullDescription
      mask DialogControl n Prompt: Number of columns in matrix A
  Real-Imag to Complex : RealImagToComplex
  State Control : StateControl  StateControl=Synchronous
  Unit Delay Enabled Synchronous1 : hdlsllib/Discrete/Unit Delay Enabled Synchronous  InitialCondition=0.0  SampleTime=-1
      settings: SourceProductBaseCode=SL
  Unit Delay Enabled Synchronous3 : hdlsllib/Discrete/Unit Delay Enabled Synchronous  InitialCondition=0.0  SampleTime=-1
      settings: SourceProductBaseCode=SL
  ValidIn to Ready Logic : Subsystem
  ValidIn to Ready Logic1 : Subsystem
  xOut : Outport  VectorParamsAs1DForOutWhenUnconnected=off
  validOut : Outport  Port=2  VectorParamsAs1DForOutWhenUnconnected=off
  ready : Outport  Port=3  VectorParamsAs1DForOutWhenUnconnected=off
  wires:
  Q-less QR Real Row Rotations/2(yOut) -> Real-Imag to Complex/2
  Q-less QR Real Row Rotations/1(xOut) -> Real-Imag to Complex/1
  Complex to Real-Imag/2 -> Q-less QR Real Row Rotations/2(y)
  Complex to Real-Imag/1 -> Q-less QR Real Row Rotations/1(x)
  restart/1 -> Q-less QR Real Row Rotations/4(restart)
  ValidIn to Ready Logic1/1(readyOut) -> ready/1
  ValidIn to Ready Logic/1(readyOut) -> ValidIn to Ready Logic1/1(readyIn)
  Q-less QR Real Row Rotations/4(ready) -> ValidIn to Ready Logic/1(readyIn)
  Q-less QR Real Row Rotations/3(validOut) -> Delay15/1, Unit Delay Enabled Synchronous3/2
  Delay9/1 -> ValidIn to Ready Logic/2(validIn), Q-less QR Real Row Rotations/3(validIn)
  x/1 -> Unit Delay Enabled Synchronous1/1
  validIn/1 -> ValidIn to Ready Logic1/2(validIn), Delay9/1, Unit Delay Enabled Synchronous1/2
  Delay15/1 -> validOut/1
  Unit Delay Enabled Synchronous1/1 -> Complex to Real-Imag/1
  Real-Imag to Complex/1 -> Unit Delay Enabled Synchronous3/1
  Unit Delay Enabled Synchronous3/1 -> xOut/1

== system qless_forgetting_factor_16x16_nofifo/MVDR_QLess_HDL/Complex Partial-Systolic Matrix Solve Using Q-less QR Decomposition with Forgetting Factor Manually Tiled n=16/Complex Partial-Systolic Q-less QR with Forgetting Factor/Complex Partial-Systolic Q-less QR with Forgetting Factor Manually tiled/Complex Partial-Systolic Q-less QR Decomposition with Forgetting Factor Section Constant pivot8/Complex Partial-Systolic Q-less QR Row Rotations/Set Element To Zero1 ==
  u : Inport
  Set Element To Zero : MATLAB Function  TreatAsAtomicUnit=on
  y : Outport  VectorParamsAs1DForOutWhenUnconnected=off
  wires:
  Set Element To Zero/1(y) -> y/1
  u/1 -> Set Element To Zero/1(u)

== system qless_forgetting_factor_16x16_nofifo/MVDR_QLess_HDL/Complex Partial-Systolic Matrix Solve Using Q-less QR Decomposition with Forgetting Factor Manually Tiled n=16/Complex Partial-Systolic Q-less QR with Forgetting Factor/Complex Partial-Systolic Q-less QR with Forgetting Factor Manually tiled/Complex Partial-Systolic Q-less QR Decomposition with Forgetting Factor Section Constant pivot8/Complex Partial-Systolic Q-less QR Row Rotations/ValidIn to Ready Logic ==
  readyIn : Inport
  validIn : Inport  Port=2
  AND : Logic  IconShape=distinctive  AllPortsSameDT=off  OutDataTypeStr=boolean
  NOT : Logic  Operator=NOT  IconShape=distinctive  AllPortsSameDT=off  OutDataTypeStr=boolean
  readyOut : Outport  VectorParamsAs1DForOutWhenUnconnected=off
  wires:
  validIn/1 -> NOT/1
  readyIn/1 -> AND/1
  AND/1 -> readyOut/1
  NOT/1 -> AND/2

== system qless_forgetting_factor_16x16_nofifo/MVDR_QLess_HDL/Complex Partial-Systolic Matrix Solve Using Q-less QR Decomposition with Forgetting Factor Manually Tiled n=16/Complex Partial-Systolic Q-less QR with Forgetting Factor/Complex Partial-Systolic Q-less QR with Forgetting Factor Manually tiled/Complex Partial-Systolic Q-less QR Decomposition with Forgetting Factor Section Constant pivot8/Complex Partial-Systolic Q-less QR Row Rotations/ValidIn to Ready Logic1 ==
  readyIn : Inport
  validIn : Inport  Port=2
  AND : Logic  IconShape=distinctive  AllPortsSameDT=off  OutDataTypeStr=boolean
  NOT : Logic  Operator=NOT  IconShape=distinctive  AllPortsSameDT=off  OutDataTypeStr=boolean
  readyOut : Outport  VectorParamsAs1DForOutWhenUnconnected=off
  wires:
  validIn/1 -> NOT/1
  readyIn/1 -> AND/1
  AND/1 -> readyOut/1
  NOT/1 -> AND/2

== system qless_forgetting_factor_16x16_nofifo/MVDR_QLess_HDL/Complex Partial-Systolic Matrix Solve Using Q-less QR Decomposition with Forgetting Factor Manually Tiled n=16/Complex Partial-Systolic Q-less QR with Forgetting Factor/Complex Partial-Systolic Q-less QR with Forgetting Factor Manually tiled/Complex Partial-Systolic Q-less QR Decomposition with Forgetting Factor Section Constant pivot9/Complex Partial-Systolic Q-less QR Row Rotations/Complex Partial-Systolic Q-less QR CORDIC Row Rotation ==
  x : Inport
  y : Inport  Port=2
  validIn : Inport  Port=3
  restart : Inport  Port=4
  CORDIC QR Kernel : MATLAB Function  TreatAsAtomicUnit=on
  Delay{1..3,6} (4 alike) : Delay  DelayLength=1
  State Control : StateControl  StateControl=Synchronous
  Unit Delay Enabled Synchronous1 : hdlsllib/Discrete/Unit Delay Enabled Synchronous  InitialCondition=0.0  SampleTime=-1
      settings: SourceProductBaseCode=SL
  Unit Delay Enabled Synchronous4 : hdlsllib/Discrete/Unit Delay Enabled Synchronous  InitialCondition=0.0  SampleTime=-1
      settings: SourceProductBaseCode=SL
  xOut : Outport  VectorParamsAs1DForOutWhenUnconnected=off
  yOut : Outport  Port=2  VectorParamsAs1DForOutWhenUnconnected=off
  validOut : Outport  Port=3  VectorParamsAs1DForOutWhenUnconnected=off
  ready : Outport  Port=4  VectorParamsAs1DForOutWhenUnconnected=off
  wires:
  Delay3/1 -> validOut/1
  Unit Delay Enabled Synchronous1/1 -> yOut/1
  CORDIC QR Kernel/1(xOut) -> Unit Delay Enabled Synchronous4/1
  y/1 -> Delay2/1
  x/1 -> Delay1/1
  CORDIC QR Kernel/2(yOut) -> Unit Delay Enabled Synchronous1/1
  validIn/1 -> Delay6/1
  Unit Delay Enabled Synchronous4/1 -> xOut/1
  restart/1 -> CORDIC QR Kernel/4(restart)
  CORDIC QR Kernel/3(validOut) -> Delay3/1, Unit Delay Enabled Synchronous4/2, Unit Delay Enabled Synchronous1/2
  CORDIC QR Kernel/4(ready) -> ready/1
  Delay1/1 -> CORDIC QR Kernel/1(xIn)
  Delay2/1 -> CORDIC QR Kernel/2(yIn)
  Delay6/1 -> CORDIC QR Kernel/3(validIn)

== system qless_forgetting_factor_16x16_nofifo/MVDR_QLess_HDL/Complex Partial-Systolic Matrix Solve Using Q-less QR Decomposition with Forgetting Factor Manually Tiled n=16/Complex Partial-Systolic Q-less QR with Forgetting Factor/Complex Partial-Systolic Q-less QR with Forgetting Factor Manually tiled/Complex Partial-Systolic Q-less QR Decomposition with Forgetting Factor Section Constant pivot9/Complex Partial-Systolic Q-less QR Row Rotations/Inverse CORDIC Gain1 ==
  u : Inport
  MATLAB Function : MATLAB Function  TreatAsAtomicUnit=on
  y : Outport  VectorParamsAs1DForOutWhenUnconnected=off
  wires:
  MATLAB Function/1(y) -> y/1
  u/1 -> MATLAB Function/1(u)

== system qless_forgetting_factor_16x16_nofifo/MVDR_QLess_HDL/Complex Partial-Systolic Matrix Solve Using Q-less QR Decomposition with Forgetting Factor Manually Tiled n=16/Complex Partial-Systolic Q-less QR with Forgetting Factor/Complex Partial-Systolic Q-less QR with Forgetting Factor Manually tiled/Complex Partial-Systolic Q-less QR Decomposition with Forgetting Factor Section Constant pivot9/Complex Partial-Systolic Q-less QR Row Rotations/Inverse CORDIC Gain4 ==
  u : Inport
  MATLAB Function : MATLAB Function  TreatAsAtomicUnit=on
  y : Outport  VectorParamsAs1DForOutWhenUnconnected=off
  wires:
  MATLAB Function/1(y) -> y/1
  u/1 -> MATLAB Function/1(u)

== system qless_forgetting_factor_16x16_nofifo/MVDR_QLess_HDL/Complex Partial-Systolic Matrix Solve Using Q-less QR Decomposition with Forgetting Factor Manually Tiled n=16/Complex Partial-Systolic Q-less QR with Forgetting Factor/Complex Partial-Systolic Q-less QR with Forgetting Factor Manually tiled/Complex Partial-Systolic Q-less QR Decomposition with Forgetting Factor Section Constant pivot9/Complex Partial-Systolic Q-less QR Row Rotations/Q-less QR Rotate First Element To Real1 ==
  x : Inport
  validIn : Inport  Port=2
  restart : Inport  Port=3
  Complex to Real-Imag : ComplexToRealImag
  Delay15 : Delay  DelayLength=1
  Delay9 : Delay  DelayLength=1
  Q-less QR Real Row Rotations : Subsystem  mask(QR Real Row Rotations){n=n, pivot=pivot}
      mask prompts: n "fixed:emblib:ColumnsInA"
      mask help: fixed:emblib:RowRotationsFullDescription
      mask DialogControl n Prompt: Number of columns in matrix A
  Real-Imag to Complex : RealImagToComplex
  State Control : StateControl  StateControl=Synchronous
  Unit Delay Enabled Synchronous1 : hdlsllib/Discrete/Unit Delay Enabled Synchronous  InitialCondition=0.0  SampleTime=-1
      settings: SourceProductBaseCode=SL
  Unit Delay Enabled Synchronous3 : hdlsllib/Discrete/Unit Delay Enabled Synchronous  InitialCondition=0.0  SampleTime=-1
      settings: SourceProductBaseCode=SL
  ValidIn to Ready Logic : Subsystem
  ValidIn to Ready Logic1 : Subsystem
  xOut : Outport  VectorParamsAs1DForOutWhenUnconnected=off
  validOut : Outport  Port=2  VectorParamsAs1DForOutWhenUnconnected=off
  ready : Outport  Port=3  VectorParamsAs1DForOutWhenUnconnected=off
  wires:
  Q-less QR Real Row Rotations/2(yOut) -> Real-Imag to Complex/2
  Q-less QR Real Row Rotations/1(xOut) -> Real-Imag to Complex/1
  Complex to Real-Imag/2 -> Q-less QR Real Row Rotations/2(y)
  Complex to Real-Imag/1 -> Q-less QR Real Row Rotations/1(x)
  restart/1 -> Q-less QR Real Row Rotations/4(restart)
  ValidIn to Ready Logic1/1(readyOut) -> ready/1
  ValidIn to Ready Logic/1(readyOut) -> ValidIn to Ready Logic1/1(readyIn)
  Q-less QR Real Row Rotations/4(ready) -> ValidIn to Ready Logic/1(readyIn)
  Q-less QR Real Row Rotations/3(validOut) -> Delay15/1, Unit Delay Enabled Synchronous3/2
  Delay9/1 -> ValidIn to Ready Logic/2(validIn), Q-less QR Real Row Rotations/3(validIn)
  x/1 -> Unit Delay Enabled Synchronous1/1
  validIn/1 -> ValidIn to Ready Logic1/2(validIn), Delay9/1, Unit Delay Enabled Synchronous1/2
  Delay15/1 -> validOut/1
  Unit Delay Enabled Synchronous1/1 -> Complex to Real-Imag/1
  Real-Imag to Complex/1 -> Unit Delay Enabled Synchronous3/1
  Unit Delay Enabled Synchronous3/1 -> xOut/1

== system qless_forgetting_factor_16x16_nofifo/MVDR_QLess_HDL/Complex Partial-Systolic Matrix Solve Using Q-less QR Decomposition with Forgetting Factor Manually Tiled n=16/Complex Partial-Systolic Q-less QR with Forgetting Factor/Complex Partial-Systolic Q-less QR with Forgetting Factor Manually tiled/Complex Partial-Systolic Q-less QR Decomposition with Forgetting Factor Section Constant pivot9/Complex Partial-Systolic Q-less QR Row Rotations/Set Element To Zero1 ==
  u : Inport
  Set Element To Zero : MATLAB Function  TreatAsAtomicUnit=on
  y : Outport  VectorParamsAs1DForOutWhenUnconnected=off
  wires:
  Set Element To Zero/1(y) -> y/1
  u/1 -> Set Element To Zero/1(u)
